simulink model "para_estimation"  (R2022b)
settings: Solver=FixedStepAuto  StartTime=0.0  StopTime=10.0  FixedStep=Ts  RelTol=1e-3
values from neighbouring files (symbols this model uses):
  z_initial = [theta(1); x(1); y(1)]    [Run_model.m]
settings Model: Creator=digitalstorm  LastModifiedBy=digitalstorm

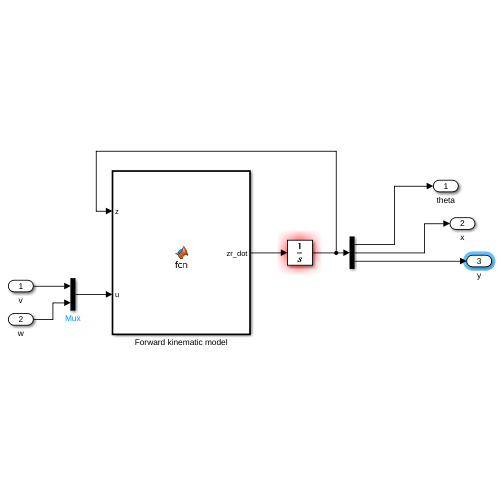
[thumbnail: Simulink's stored preview of the top-level diagram]
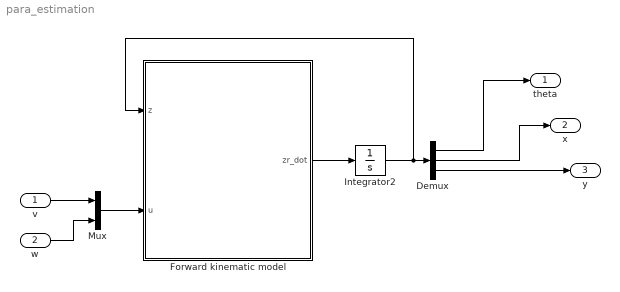
== system para_estimation ==
  v : Inport
  w : Inport  Port=2
  Demux : Demux  Outputs=3
  Forward kinematic model : MATLAB Function  TreatAsAtomicUnit=on
  Integrator2 : Integrator  InitialCondition=z_initial
  Mux : Mux  Inputs=2
  theta : Outport
  x : Outport  Port=2
  y : Outport  Port=3
  wires:
  Integrator2/1 -> Demux/1, Forward kinematic model/1(z)
  Forward kinematic model/1(zr_dot) -> Integrator2/1
  Mux/1 -> Forward kinematic model/2(u)
  v/1 -> Mux/1
  w/1 -> Mux/2
  Demux/1 -> theta/1
  Demux/2 -> x/1
  Demux/3 -> y/1

== matlab function para_estimation/Forward kinematic model ==
  data: z input; u input; zr_dot output; d parameter
function zr_dot = fcn(z,u,d)

%% unpacking the state vectors
theta=z(1);

%% unpacking the intput
v=u(1);
omega=u(2);

%% ODE
theta_dot=omega;
x_dot=v*cos(theta)-d*omega*sin(theta);
y_dot=v*sin(theta)+d*omega*cos(theta);
% phir_dot = (v+omega)/r;
% phil_dot = (v-omega)/r;


%% packing the output
zr_dot=[theta_dot;x_dot;y_dot];
